simulink library "Yaw_System_Lib"  (Simulink 7.9)
settings: Solver=ode45  StartTime=0.0  StopTime=10.0  RelTol=1e-3
undefined symbols (not defined in the file): WT_Params
libraries: mblibv1 x45, Yaw_Actuation_Lib x3, Yaw_System_Lib x1
(part 1 of 2)
Description:
  | Copyright 2011 MathWorks, Inc.
settings Model: Creator=smiller  LastModifiedBy=smiller

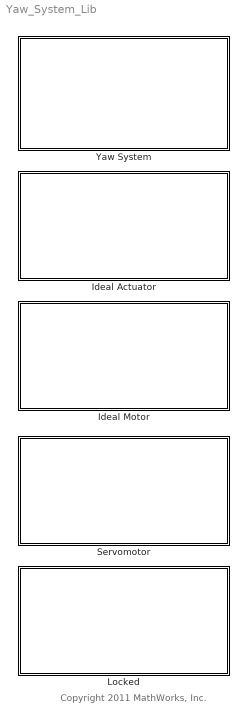
== system Yaw_System_Lib ==
  note: Copyright 2011 MathWorks, Inc.
  Ideal Actuator : Subsystem
      mask Display: image(imread('Yaw_Ideal_Actuator_System_IMAGE.jpg'));
  Ideal Motor : Subsystem
      mask Display: image(imread('Yaw_Ideal_Motor_System_IMAGE.jpg'));
  Locked : Subsystem
      mask Display: image(imread('Yaw_Locked_System_IMAGE.jpg'));
  Servomotor : Subsystem
      mask Display: image(imread('Yaw_Servomotor_System_IMAGE.jpg'));
  Yaw System : Subsystem  BlockChoice=Ideal Actuator
      settings: TemplateBlock=self  MemberBlocks=Ideal Actuator,Ideal Motor,Locked,Servomotor

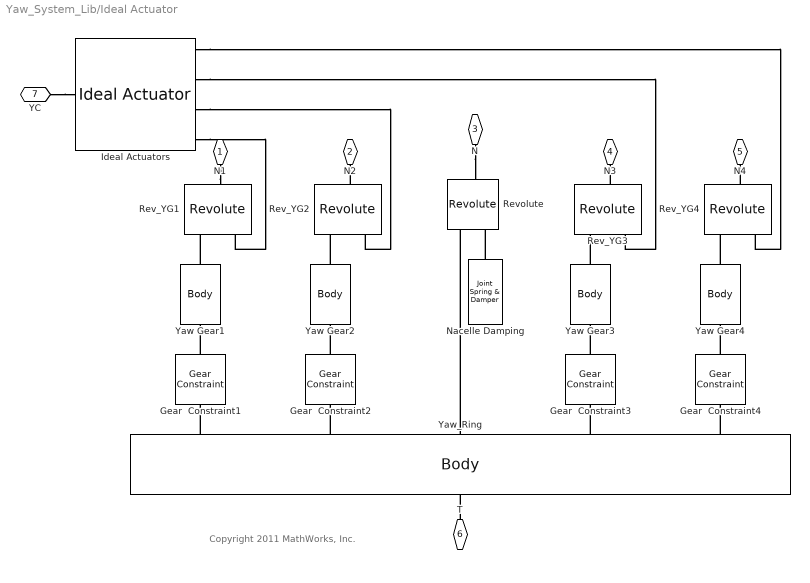
== system Yaw_System_Lib/Ideal Actuator ==
  note: Copyright 2011 MathWorks, Inc.
  Gear  Constraint{1..4} (4 alike) : mblibv1/Constraints &  Drivers/Gear Constraint  PhysicalDomain=mechanical  SubClassName=Unknown  LeftPortType=blob  RightPortType=blob  LConnTagsString=__newl0  RConnTagsString=__newr0  UpdateFromCAD=off  DialogClass=GearConstraint  NumSAPorts=0  BaseRadius=WT_Params.Yaw_Actuator.yaw_ring_diameter/2  BaseRadiusUnits=m  FollowerRadius=WT_Params.Yaw_Actuator.yaw_gear_diameter/2  FollowerRadiusUnits=m
  Ideal Actuators : Yaw_Actuation_Lib/Ideal Actuator  SystemSampleTime=-1
  Nacelle Damping : mblibv1/Force  Elements/Joint Spring & Damper  SystemSampleTime=-1  UpdateFromCAD=off  DialogClass=JointSpringDamper  JFEParameters=P1$false$0$0$0$m$m/s$N$deg$deg/s$N*m#P2$false$0$0$0$m$m/s$N$deg$deg/s$N*m#P3$false$0$0$0$m$m/s$N$deg$deg/s$N*m#R1$true$0$WT_Params.Nacelle.damping$0$m$m/s$N$deg$deg/s$N*m#R2$false$0$0$0$m$m/s$N$deg$deg/s$N*m#R3$false$0$0$0$m$m/s$N$deg$deg/s$N*m#S$false$0$0$0$m$m/s$N$deg$deg/s$N*m
  Rev_YG{1..4} (4 alike) : mblibv1/Joints/Revolute  LConnTagsString=__newl0|SA1  RConnTagsString=__newr0  UpdateFromCAD=off  NumSAPorts=1  CutJoint=off  MarkAsCut=off  Primitives=prismatic  PrimitiveProps=R1$Base$[0 1 0]$revolute  DialogClass=JointBlock  R1Axis=[0 1 0]
  Revolute : mblibv1/Joints/Revolute  LConnTagsString=__newl0|SA1  RConnTagsString=__newr0  UpdateFromCAD=off  NumSAPorts=1  CutJoint=off  MarkAsCut=off  Primitives=prismatic  PrimitiveProps=R1$Base$[0 1 0]$revolute  DialogClass=JointBlock  R1Axis=[0 1 0]
  Yaw Gear{1..4} (4 alike) : mblibv1/Bodies/Body  PhysicalDomain=mechanical  SubClassName=Unknown  LeftPortType=workingframe  RightPortType=workingframe  LConnTagsString=CG  RConnTagsString=CS1  UpdateFromCAD=off  DialogClass=MechanicalBodyBlock  Mass=1  MassUnits=kg  InertiaUnits=kg*m^2  Inertia=eye(3)  Shape=Cylinder  ShapeDims=[1 1]  ShapeUnits=m  ShapeUse=false  Density=1  DensityUnits=kg/m^3  DensityUse=false  GraphicsMode=MACHINE_DEFAULT  BodyColorSelMode=COLORPALETTE  BodyColor=[0 0 1]  AttachedToCS=CG  CG=Left$CG$[0 0 0]$ADJOINING$ADJOINING$m$[0 0 0]$Euler X-Y-Z$deg$ADJOINING$true$none  WorkingFrames=Right$CS1$[0 0 0]$CG$CG$m$[0 0 0]$Euler X-Y-Z$deg$CG$true$none#Right$CS5$[0 0 0]$CG$CG$m$[0 0 0]$Euler X-Y-Z$deg$CG$false$none#Right$CS7$[WT_Params.Yaw_Actuator.yaw_gear_diameter/2*cos(0) -0.5*WT_Params.Yaw_Actuator.yaw_gear_thickness WT_Params.Yaw_Actuator.yaw_gear_diameter/2*sin(0)]$CG$CG$m$[0 0 0]$Euler X-Y-Z$deg$CG$false$none#Right$CS17$[WT_Params.Yaw_Actuator.yaw_gear_diameter/2*cos(0) 0.5*WT_Params.Yaw_Actuator.yaw_gear_thickness WT_Params.Yaw_Actuator.yaw_gear_diameter/2*sin(0)]$CG$CG$m$[0 0 0]$Euler X-Y-Z$deg$CG$false$none#Right$CS8$[WT_Params.Yaw_Actuator.yaw_gear_diameter/2*cos(0.2*pi) -0.5*WT_Params.Yaw_Actuator.yaw_gear_thickness WT_Params.Yaw_Actuator.yaw_gear_diameter/2*sin(0.2*pi)]$CG$CG$m$[0 0 0]$Euler X-Y-Z$deg$CG$false$none#Right$CS18$[WT_Params.Yaw_Actuator.yaw_gear_diameter/2*cos(0.2*pi) 0.5*WT_Params.Yaw_Actuator.yaw_gear_thickness WT_Params.Yaw_Actuator.yaw_gear_diameter/2*sin(0.2*pi)]$CG$CG$m$[0 0 0]$Euler X-Y-Z$deg$CG$false$none#Right$CS9$[WT_Params.Yaw_Actuator.yaw_gear_diameter/2*cos(0.4*pi) -0.5*WT_Params.Yaw_Actuator.yaw_gear_thickness WT_Params.Yaw_Actuator.yaw_gear_diameter/2*sin(0.4*pi)]$CG$CG$m$[0 0 0]$Euler X-Y-Z$deg$CG$false$none#Right$CS19$[WT_Params.Yaw_Actuator.yaw_gear_diameter/2*cos(0.4*pi) 0.5*WT_Params.Yaw_Actuator.yaw_gear_thickness WT_Params.Yaw_Actuator.yaw_gear_diameter/2*sin(0.4*pi)]$CG$CG$m$[0 0 0]$Euler X-Y-Z$deg$CG$false$none#Right$CS10$[WT_Params.Yaw_Actuator.yaw_gear_diameter/2*cos(0.6*pi) -0.5*WT_Params.Yaw_Actuator.yaw_gear_thickness WT_Params.Yaw_Actuator.yaw_gear_diameter/2*sin(0.6*pi)]$CG$CG$m$[0 0 0]$Euler X-Y-Z$deg$CG$false$none#Right$CS20$[WT_Params.Yaw_Actuator.yaw_gear_diameter/2*cos(0.6*pi) 0.5*WT_Params.Yaw_Actuator.yaw_gear_thickness WT_Params.Yaw_Actuator.yaw_gear_diameter/2*sin(0.6*pi)]$CG$CG$m$[0 0 0]$Euler X-Y-Z$deg$CG$false$none#Right$CS11$[WT_Params.Yaw_Actuator.yaw_gear_diameter/2*cos(0.8*pi) -0.5*WT_Params.Yaw_Actuator.yaw_gear_thickness WT_Params.Yaw_Actuator.yaw_gear_diameter/2*sin(0.8*pi)]$CG$CG$m$[0 0 0]$Euler X-Y-Z$deg$CG$false$none#Right$CS21$[WT_Params.Yaw_Actuator.yaw_gear_diameter/2*cos(0.8*pi) 0.5*WT_Params.Yaw_Actuator.yaw_gear_thickness WT_Params.Yaw_Actuator.yaw_gear_diameter/2*sin(0.8*pi)]$CG$CG$m$[0 0 0]$Euler X-Y-Z$deg$CG$false$none#Right$CS12$[WT_Params.Yaw_Actuator.yaw_gear_diameter/2*cos(1.0*pi) -0.5*WT_Params.Yaw_Actuator.yaw_gear_thickness WT_Params.Yaw_Actuator.yaw_gear_diameter/2*sin(1.0*pi)]$CG$CG$m$[0 0 0]$Euler X-Y-Z$deg$CG$false$none#Right$CS22$[WT_Params.Yaw_Actuator.yaw_gear_diameter/2*cos(1.0*pi) 0.5*WT_Params.Yaw_Actuator.yaw_gear_thickness WT_Params.Yaw_Actuator.yaw_gear_diameter/2*sin(1.0*pi)]$CG$CG$m$[0 0 0]$Euler X-Y-Z$deg$CG$false$none#Right$CS13$[WT_Params.Yaw_Actuator.yaw_gear_diameter/2*cos(1.2*pi) -0.5*WT_Params.Yaw_Actuator.yaw_gear_thickness WT_Params.Yaw_Actuator.yaw_gear_diameter/2*sin(1.2*pi)]$CG$CG$m$[0 0 0]$Euler X-Y-Z$deg$CG$false$none#Right$CS23$[WT_Params.Yaw_Actuator.yaw_gear_diameter/2*cos(1.2*pi) 0.5*WT_Params.Yaw_Actuator.yaw_gear_thickness WT_Params.Yaw_Actuator.yaw_gear_diameter/2*sin(1.2*pi)]$CG$CG$m$[0 0 0]$Euler X-Y-Z$deg$CG$false$none#Right$CS14$[WT_Params.Yaw_Actuator.yaw_gear_diameter/2*cos(1.4*pi) -0.5*WT_Params.Yaw_Actuator.yaw_gear_thickness WT_Params.Yaw_Actuator.yaw_gear_diameter/2*sin(1.4*pi)]$CG$CG$m$[0 0 0]$Euler X-Y-Z$deg$CG$false$none#Right$CS24$[WT_Params.Yaw_Actuator.yaw_gear_diameter/2*cos(1.4*pi) 0.5*WT_Params.Yaw_Actuator.yaw_gear_thickness WT_Params.Yaw_Actuator.yaw_gear_diameter/2*sin(1.4*pi)]$CG$CG$m$[0 0 0]$Euler X-Y-Z$deg$CG$false$none#Right$CS15$[WT_Params.Yaw_Actuator.yaw_gear_diameter/2*cos(1.6*pi) -0.5*WT_Params.Yaw_Actuator.yaw_gear_thickness WT_Params.Yaw_Actuator.yaw_gear_diameter/2*sin(1.6*pi)]$CG$CG$m$[0 0 0]$Euler X-Y-Z$deg$CG$false$none#Right$CS25$[WT_Params.Yaw_Actuator.yaw_gear_diameter/2*cos(1.6*pi) 0.5*WT_Params.Yaw_Actuator.yaw_gear_thickness WT_Params.Yaw_Actuator.yaw_gear_diameter/2*sin(1.6*pi)]$CG$CG$m$[0 0 0]$Euler X-Y-Z$deg$CG$false$none#Right$CS16$[WT_Params.Yaw_Actuator.yaw_gear_diameter/2*cos(1.8*pi) -0.5*WT_Params.Yaw_Actuator.yaw_gear_thickness WT_Params.Yaw_Actuator.yaw_gear_diameter/2*sin(1.8*pi)]$CG$CG$m$[0 0 0]$Euler X-Y-Z$deg$CG$false$none#Right$CS26$[WT_Params.Yaw_Actuator.yaw_gear_diameter/2*cos(1.8*pi) 0.5*WT_Params.Yaw_Actuator.yaw_gear_thickness WT_Params.Yaw_Actuator.yaw_gear_diameter/2*sin(1.8*pi)]$CG$CG$m$[0 0 0]$Euler X-Y-Z$deg$CG$false$none  CGPos=[0 0 0]  CGRot=[0 0 0]  CS0Pos=[]  CS0Rot=[]  CS1Pos=[0 0 0]  CS1Rot=[0 0 0]  CS2Pos=[]  CS2Rot=[]  CS3Pos=[]  CS3Rot=[]  CS4Pos=[]  CS4Rot=[]  CS5Pos=[0 0 0]  CS5Rot=[0 0 0]  CS6Pos=[]  CS6Rot=[]  CS7Pos=[WT_Params.Yaw_Actuator.yaw_gear_diameter/2*cos(0) -0.5*WT_Params.Yaw_Actuator.yaw_gear_thickness WT_Params.Yaw_Actuator.yaw_gear_diameter/2*sin(0)]  CS7Rot=[0 0 0]  CS8Pos=[WT_Params.Yaw_Actuator.yaw_gear_diameter/2*cos(0.2*pi) -0.5*WT_Params.Yaw_Actuator.yaw_gear_thickness WT_Params.Yaw_Actuator.yaw_gear_diameter/2*sin(0.2*pi)]  CS8Rot=[0 0 0]  CS9Pos=[WT_Params.Yaw_Actuator.yaw_gear_diameter/2*cos(0.4*pi) -0.5*WT_Params.Yaw_Actuator.yaw_gear_thickness WT_Params.Yaw_Actuator.yaw_gear_diameter/2*sin(0.4*pi)]  CS9Rot=[0 0 0]  CS10Pos=[WT_Params.Yaw_Actuator.yaw_gear_diameter/2*cos(0.6*pi) -0.5*WT_Params.Yaw_Actuator.yaw_gear_thickness WT_Params.Yaw_Actuator.yaw_gear_diameter/2*sin(0.6*pi)]  CS10Rot=[0 0 0]  CS11Pos=[WT_Params.Yaw_Actuator.yaw_gear_diameter/2*cos(0.8*pi) -0.5*WT_Params.Yaw_Actuator.yaw_gear_thickness WT_Params.Yaw_Actuator.yaw_gear_diameter/2*sin(0.8*pi)]  CS11Rot=[0 0 0]  CS12Pos=[WT_Params.Yaw_Actuator.yaw_gear_diameter/2*cos(1.0*pi) -0.5*WT_Params.Yaw_Actuator.yaw_gear_thickness WT_Params.Yaw_Actuator.yaw_gear_diameter/2*sin(1.0*pi)]  CS12Rot=[0 0 0]  CS13Pos=[WT_Params.Yaw_Actuator.yaw_gear_diameter/2*cos(1.2*pi) -0.5*WT_Params.Yaw_Actuator.yaw_gear_thickness WT_Params.Yaw_Actuator.yaw_gear_diameter/2*sin(1.2*pi)]  CS13Rot=[0 0 0]  CS14Pos=[WT_Params.Yaw_Actuator.yaw_gear_diameter/2*cos(1.4*pi) -0.5*WT_Params.Yaw_Actuator.yaw_gear_thickness WT_Params.Yaw_Actuator.yaw_gear_diameter/2*sin(1.4*pi)]  CS14Rot=[0 0 0]  CS15Pos=[WT_Params.Yaw_Actuator.yaw_gear_diameter/2*cos(1.6*pi) -0.5*WT_Params.Yaw_Actuator.yaw_gear_thickness WT_Params.Yaw_Actuator.yaw_gear_diameter/2*sin(1.6*pi)]  CS15Rot=[0 0 0]  CS16Pos=[WT_Params.Yaw_Actuator.yaw_gear_diameter/2*cos(1.8*pi) -0.5*WT_Params.Yaw_Actuator.yaw_gear_thickness WT_Params.Yaw_Actuator.yaw_gear_diameter/2*sin(1.8*pi)]  CS16Rot=[0 0 0]  CS17Pos=[WT_Params.Yaw_Actuator.yaw_gear_diameter/2*cos(0) 0.5*WT_Params.Yaw_Actuator.yaw_gear_thickness WT_Params.Yaw_Actuator.yaw_gear_diameter/2*sin(0)]  CS17Rot=[0 0 0]  CS18Pos=[WT_Params.Yaw_Actuator.yaw_gear_diameter/2*cos(0.2*pi) 0.5*WT_Params.Yaw_Actuator.yaw_gear_thickness WT_Params.Yaw_Actuator.yaw_gear_diameter/2*sin(0.2*pi)]  CS18Rot=[0 0 0]  CS19Pos=[WT_Params.Yaw_Actuator.yaw_gear_diameter/2*cos(0.4*pi) 0.5*WT_Params.Yaw_Actuator.yaw_gear_thickness WT_Params.Yaw_Actuator.yaw_gear_diameter/2*sin(0.4*pi)]  CS19Rot=[0 0 0]  CS20Pos=[WT_Params.Yaw_Actuator.yaw_gear_diameter/2*cos(0.6*pi) 0.5*WT_Params.Yaw_Actuator.yaw_gear_thickness WT_Params.Yaw_Actuator.yaw_gear_diameter/2*sin(0.6*pi)]  CS20Rot=[0 0 0]
  Yaw_Ring : mblibv1/Bodies/Body  LConnTagsString=CS3|CS4|CS2|CS6|CS27  RConnTagsString=CS1  UpdateFromCAD=off  DialogClass=MechanicalBodyBlock  Mass=1  MassUnits=kg  InertiaUnits=kg*m^2  Inertia=eye(3)  Shape=Cylinder  ShapeDims=[1 1]  ShapeUnits=m  ShapeUse=false  Density=1  DensityUnits=kg/m^3  DensityUse=false  GraphicsMode=MACHINE_DEFAULT  BodyColorSelMode=COLORPALETTE  BodyColor=[0.74902 0.74902 0]  AttachedToCS=CG  CG=Left$CG$[0 0 0]$CS1$CS1$m$[0 0 0]$Euler X-Y-Z$deg$CS1$false$none  WorkingFrames=Left$CS3$[0 0 0]$CS1$CS1$m$[0 0 0]$Euler X-Y-Z$deg$CS1$true$none#Left$CS4$[0 0 0]$CS1$CS1$m$[0 0 0]$Euler X-Y-Z$deg$CS1$true$none#Left$CS2$[0 0 0]$CS1$CS1$m$[0 0 0]$Euler X-Y-Z$deg$CS1$true$none#Left$CS6$[0 0 0]$CS1$CS1$m$[0 0 0]$Euler X-Y-Z$deg$CS1$true$none#Left$CS27$[0 0 0]$CS1$CS1$m$[0 0 0]$Euler X-Y-Z$deg$CS1$true$none#Right$CS1$[0 0 0]$Adjoining$Adjoining$m$[0 0 0]$Euler X-Y-Z$deg$Adjoining$true$none#Right$CS5$[0 0 0]$CG$CG$m$[0 0 0]$Euler X-Y-Z$deg$CG$false$none#Right$CS7$[WT_Params.Yaw_Actuator.yaw_ring_diameter/2*cos(0) -0.5*WT_Params.Yaw_Actuator.yaw_ring_thickness WT_Params.Yaw_Actuator.yaw_ring_diameter/2*sin(0)]$CG$CG$m$[0 0 0]$Euler X-Y-Z$deg$CG$false$none#Right$CS17$[WT_Params.Yaw_Actuator.yaw_ring_diameter/2*cos(0) 0.5*WT_Params.Yaw_Actuator.yaw_gear_thickness WT_Params.Yaw_Actuator.yaw_ring_diameter/2*sin(0)]$CG$CG$m$[0 0 0]$Euler X-Y-Z$deg$CG$false$none#Right$CS8$[WT_Params.Yaw_Actuator.yaw_ring_diameter/2*cos(0.2*pi) -0.5*WT_Params.Yaw_Actuator.yaw_gear_thickness WT_Params.Yaw_Actuator.yaw_ring_diameter/2*sin(0.2*pi)]$CG$CG$m$[0 0 0]$Euler X-Y-Z$deg$CG$false$none#Right$CS18$[WT_Params.Yaw_Actuator.yaw_ring_diameter/2*cos(0.2*pi) 0.5*WT_Params.Yaw_Actuator.yaw_ring_thickness WT_Params.Yaw_Actuator.yaw_ring_diameter/2*sin(0.2*pi)]$CG$CG$m$[0 0 0]$Euler X-Y-Z$deg$CG$false$none#Right$CS9$[WT_Params.Yaw_Actuator.yaw_ring_diameter/2*cos(0.4*pi) -0.5*WT_Params.Yaw_Actuator.yaw_ring_thickness WT_Params.Yaw_Actuator.yaw_ring_diameter/2*sin(0.4*pi)]$CG$CG$m$[0 0 0]$Euler X-Y-Z$deg$CG$false$none#Right$CS19$[WT_Params.Yaw_Actuator.yaw_ring_diameter/2*cos(0.4*pi) 0.5*WT_Params.Yaw_Actuator.yaw_ring_thickness WT_Params.Yaw_Actuator.yaw_ring_diameter/2*sin(0.4*pi)]$CG$CG$m$[0 0 0]$Euler X-Y-Z$deg$CG$false$none#Right$CS10$[WT_Params.Yaw_Actuator.yaw_ring_diameter/2*cos(0.6*pi) -0.5*WT_Params.Yaw_Actuator.yaw_ring_thickness WT_Params.Yaw_Actuator.yaw_ring_diameter/2*sin(0.6*pi)]$CG$CG$m$[0 0 0]$Euler X-Y-Z$deg$CG$false$none#Right$CS20$[WT_Params.Yaw_Actuator.yaw_ring_diameter/2*cos(0.6*pi) 0.5*WT_Params.Yaw_Actuator.yaw_ring_thickness WT_Params.Yaw_Actuator.yaw_ring_diameter/2*sin(0.6*pi)]$CG$CG$m$[0 0 0]$Euler X-Y-Z$deg$CG$false$none#Right$CS11$[WT_Params.Yaw_Actuator.yaw_ring_diameter/2*cos(0.8*pi) -0.5*WT_Params.Yaw_Actuator.yaw_ring_thickness WT_Params.Yaw_Actuator.yaw_ring_diameter/2*sin(0.8*pi)]$CG$CG$m$[0 0 0]$Euler X-Y-Z$deg$CG$false$none#Right$CS21$[WT_Params.Yaw_Actuator.yaw_ring_diameter/2*cos(0.8*pi) 0.5*WT_Params.Yaw_Actuator.yaw_ring_thickness WT_Params.Yaw_Actuator.yaw_ring_diameter/2*sin(0.8*pi)]$CG$CG$m$[0 0 0]$Euler X-Y-Z$deg$CG$false$none#Right$CS12$[WT_Params.Yaw_Actuator.yaw_ring_diameter/2*cos(1.0*pi) -0.5*WT_Params.Yaw_Actuator.yaw_ring_thickness WT_Params.Yaw_Actuator.yaw_gear_diameter/2*sin(1.0*pi)]$CG$CG$m$[0 0 0]$Euler X-Y-Z$deg$CG$false$none#Right$CS22$[WT_Params.Yaw_Actuator.yaw_gear_diameter/2*cos(1.0*pi) 0.5*WT_Params.Yaw_Actuator.yaw_ring_thickness WT_Params.Yaw_Actuator.yaw_ring_diameter/2*sin(1.0*pi)]$CG$CG$m$[0 0 0]$Euler X-Y-Z$deg$CG$false$none#Right$CS13$[WT_Params.Yaw_Actuator.yaw_ring_diameter/2*cos(1.2*pi) -0.5*WT_Params.Yaw_Actuator.yaw_ring_thickness WT_Params.Yaw_Actuator.yaw_ring_diameter/2*sin(1.2*pi)]$CG$CG$m$[0 0 0]$Euler X-Y-Z$deg$CG$false$none#Right$CS23$[WT_Params.Yaw_Actuator.yaw_ring_diameter/2*cos(1.2*pi) 0.5*WT_Params.Yaw_Actuator.yaw_ring_thickness WT_Params.Yaw_Actuator.yaw_ring_diameter/2*sin(1.2*pi)]$CG$CG$m$[0 0 0]$Euler X-Y-Z$deg$CG$false$none#Right$CS14$[WT_Params.Yaw_Actuator.yaw_ring_diameter/2*cos(1.4*pi) -0.5*WT_Params.Yaw_Actuator.yaw_gear_thickness WT_Params.Yaw_Actuator.yaw_ring_diameter/2*sin(1.4*pi)]$CG$CG$m$[0 0 0]$Euler X-Y-Z$deg$CG$false$none#Right$CS24$[WT_Params.Yaw_Actuator.yaw_ring_diameter/2*cos(1.4*pi) 0.5*WT_Params.Yaw_Actuator.yaw_ring_thickness WT_Params.Yaw_Actuator.yaw_ring_diameter/2*sin(1.4*pi)]$CG$CG$m$[0 0 0]$Euler X-Y-Z$deg$CG$false$none#Right$CS15$[WT_Params.Yaw_Actuator.yaw_ring_diameter/2*cos(1.6*pi) -0.5*WT_Params.Yaw_Actuator.yaw_ring_thickness WT_Params.Yaw_Actuator.yaw_ring_diameter/2*sin(1.6*pi)]$CG$CG$m$[0 0 0]$Euler X-Y-Z$deg$CG$false$none#Right$CS25$[WT_Params.Yaw_Actuator.yaw_ring_diameter/2*cos(1.6*pi) 0.5*WT_Params.Yaw_Actuator.yaw_ring_thickness WT_Params.Yaw_Actuator.yaw_ring_diameter/2*sin(1.6*pi)]$CG$CG$m$[0 0 0]$Euler X-Y-Z$deg$CG$false$none#Right$CS16$[WT_Params.Yaw_Actuator.yaw_ring_diameter/2*cos(1.8*pi) -0.5*WT_Params.Yaw_Actuator.yaw_ring_thickness WT_Params.Yaw_Actuator.yaw_ring_diameter/2*sin(1.8*pi)]$CG$CG$m$[0 0 0]$Euler X-Y-Z$deg$CG$false$none#Right$CS26$[WT_Params.Yaw_Actuator.yaw_ring_diameter/2*cos(1.8*pi) 0.5*WT_Params.Yaw_Actuator.yaw_ring_thickness WT_Params.Yaw_Actuator.yaw_ring_diameter/2*sin(1.8*pi)]$CG$CG$m$[0 0 0]$Euler X-Y-Z$deg$CG$false$none  CGPos=[0 0 0]  CGRot=[0 0 0]  CS0Pos=[]  CS0Rot=[]  CS1Pos=[0 0 0]  CS1Rot=[0 0 0]  CS2Pos=[0 0 0]  CS2Rot=[0 0 0]  CS3Pos=[0 0 0]  CS3Rot=[0 0 0]  CS4Pos=[0 0 0]  CS4Rot=[0 0 0]  CS5Pos=[0 0 0]  CS5Rot=[0 0 0]  CS6Pos=[0 0 0]  CS6Rot=[0 0 0]  CS7Pos=[WT_Params.Yaw_Actuator.yaw_ring_diameter/2*cos(0) -0.5*WT_Params.Yaw_Actuator.yaw_ring_thickness WT_Params.Yaw_Actuator.yaw_ring_diameter/2*sin(0)]  CS7Rot=[0 0 0]  CS8Pos=[WT_Params.Yaw_Actuator.yaw_ring_diameter/2*cos(0.2*pi) -0.5*WT_Params.Yaw_Actuator.yaw_gear_thickness WT_Params.Yaw_Actuator.yaw_ring_diameter/2*sin(0.2*pi)]  CS8Rot=[0 0 0]  CS9Pos=[WT_Params.Yaw_Actuator.yaw_ring_diameter/2*cos(0.4*pi) -0.5*WT_Params.Yaw_Actuator.yaw_ring_thickness WT_Params.Yaw_Actuator.yaw_ring_diameter/2*sin(0.4*pi)]  CS9Rot=[0 0 0]  CS10Pos=[WT_Params.Yaw_Actuator.yaw_ring_diameter/2*cos(0.6*pi) -0.5*WT_Params.Yaw_Actuator.yaw_ring_thickness WT_Params.Yaw_Actuator.yaw_ring_diameter/2*sin(0.6*pi)]  CS10Rot=[0 0 0]  CS11Pos=[WT_Params.Yaw_Actuator.yaw_ring_diameter/2*cos(0.8*pi) -0.5*WT_Params.Yaw_Actuator.yaw_ring_thickness WT_Params.Yaw_Actuator.yaw_ring_diameter/2*sin(0.8*pi)]  CS11Rot=[0 0 0]  CS12Pos=[WT_Params.Yaw_Actuator.yaw_ring_diameter/2*cos(1.0*pi) -0.5*WT_Params.Yaw_Actuator.yaw_ring_thickness WT_Params.Yaw_Actuator.yaw_gear_diameter/2*sin(1.0*pi)]  CS12Rot=[0 0 0]  CS13Pos=[WT_Params.Yaw_Actuator.yaw_ring_diameter/2*cos(1.2*pi) -0.5*WT_Params.Yaw_Actuator.yaw_ring_thickness WT_Params.Yaw_Actuator.yaw_ring_diameter/2*sin(1.2*pi)]  CS13Rot=[0 0 0]  CS14Pos=[WT_Params.Yaw_Actuator.yaw_ring_diameter/2*cos(1.4*pi) -0.5*WT_Params.Yaw_Actuator.yaw_gear_thickness WT_Params.Yaw_Actuator.yaw_ring_diameter/2*sin(1.4*pi)]  CS14Rot=[0 0 0]  CS15Pos=[WT_Params.Yaw_Actuator.yaw_ring_diameter/2*cos(1.6*pi) -0.5*WT_Params.Yaw_Actuator.yaw_ring_thickness WT_Params.Yaw_Actuator.yaw_ring_diameter/2*sin(1.6*pi)]  CS15Rot=[0 0 0]  CS16Pos=[WT_Params.Yaw_Actuator.yaw_ring_diameter/2*cos(1.8*pi) -0.5*WT_Params.Yaw_Actuator.yaw_ring_thickness WT_Params.Yaw_Actuator.yaw_ring_diameter/2*sin(1.8*pi)]  CS16Rot=[0 0 0]  CS17Pos=[WT_Params.Yaw_Actuator.yaw_ring_diameter/2*cos(0) 0.5*WT_Params.Yaw_Actuator.yaw_gear_thickness WT_Params.Yaw_Actuator.yaw_ring_diameter/2*sin(0)]  CS17Rot=[0 0 0]  CS18Pos=[WT_Params.Yaw_Actuator.yaw_ring_diameter/2*cos(0.2*pi) 0.5*WT_Params.Yaw_Actuator.yaw_ring_thickness WT_Params.Yaw_Actuator.yaw_ring_diameter/2*sin(0.2*pi)]  CS18Rot=[0 0 0]  CS19Pos=[WT_Params.Yaw_Actuator.yaw_ring_diameter/2*cos(0.4*pi) 0.5*WT_Params.Yaw_Actuator.yaw_ring_thickness WT_Params.Yaw_Actuator.yaw_ring_diameter/2*sin(0.4*pi)]  CS19Rot=[0 0 0]  CS20Pos=[WT_Params.Yaw_Actuator.yaw_ring_diameter/2*cos(0.6*pi) 0.5*WT_Params.Yaw_Actuator.yaw_ring_thickness WT_Params.Yaw_Actuator.yaw_ring_diameter/2*sin(0.6*pi)]  CS20Rot=[0 0 0]
  N1 : PMIOPort  Port=1  Side=Right
  N2 : PMIOPort  Port=2  Side=Right
  N : PMIOPort  Port=3  Side=Right
  N3 : PMIOPort  Port=4  Side=Right
  N4 : PMIOPort  Port=5  Side=Right
  T : PMIOPort  Port=6  Side=Left
  YC : PMIOPort  Port=7  Side=Right
  connections:
  Gear  Constraint1/RConn1 -- Yaw Gear1/RConn1
  Yaw Gear1/LConn1 -- Rev_YG1/LConn1
  N1/RConn1 -- Rev_YG1/RConn1
  Gear  Constraint2/RConn1 -- Yaw Gear2/RConn1
  Yaw Gear2/LConn1 -- Rev_YG2/LConn1
  Rev_YG2/RConn1 -- N2/RConn1
  Gear  Constraint3/RConn1 -- Yaw Gear3/RConn1
  Yaw Gear3/LConn1 -- Rev_YG3/LConn1
  Rev_YG3/RConn1 -- N3/RConn1
  Gear  Constraint4/RConn1 -- Yaw Gear4/RConn1
  Yaw_Ring/LConn5 -- Gear  Constraint4/LConn1
  Rev_YG4/RConn1 -- N4/RConn1
  Yaw Gear4/LConn1 -- Rev_YG4/LConn1
  YC/RConn1 -- Ideal Actuators/LConn1
  Ideal Actuators/RConn4 -- Rev_YG1/LConn2
  Ideal Actuators/RConn3 -- Rev_YG2/LConn2
  Ideal Actuators/RConn2 -- Rev_YG3/LConn2
  Ideal Actuators/RConn1 -- Rev_YG4/LConn2
  Nacelle Damping/LConn1 -- Revolute/LConn2
  N/RConn1 -- Revolute/RConn1
  Yaw_Ring/LConn3 -- Revolute/LConn1
  Yaw_Ring/LConn1 -- Gear  Constraint1/LConn1
  Yaw_Ring/LConn2 -- Gear  Constraint2/LConn1
  Yaw_Ring/LConn4 -- Gear  Constraint3/LConn1
  T/RConn1 -- Yaw_Ring/RConn1

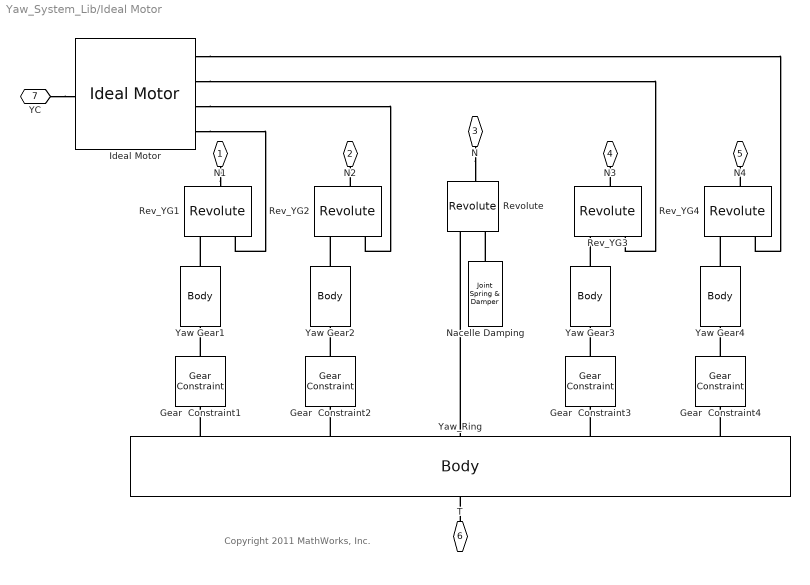
== system Yaw_System_Lib/Ideal Motor ==
  note: Copyright 2011 MathWorks, Inc.
  Gear  Constraint{1..4} (4 alike) : mblibv1/Constraints &  Drivers/Gear Constraint  PhysicalDomain=mechanical  SubClassName=Unknown  LeftPortType=blob  RightPortType=blob  LConnTagsString=__newl0  RConnTagsString=__newr0  UpdateFromCAD=off  DialogClass=GearConstraint  NumSAPorts=0  BaseRadius=WT_Params.Yaw_Actuator.yaw_ring_diameter/2  BaseRadiusUnits=m  FollowerRadius=WT_Params.Yaw_Actuator.yaw_gear_diameter/2  FollowerRadiusUnits=m
  Ideal Motor : Yaw_Actuation_Lib/Ideal Motor  SystemSampleTime=-1
  Nacelle Damping : mblibv1/Force  Elements/Joint Spring & Damper  SystemSampleTime=-1  UpdateFromCAD=off  DialogClass=JointSpringDamper  JFEParameters=P1$false$0$0$0$m$m/s$N$deg$deg/s$N*m#P2$false$0$0$0$m$m/s$N$deg$deg/s$N*m#P3$false$0$0$0$m$m/s$N$deg$deg/s$N*m#R1$true$0$WT_Params.Nacelle.damping$0$m$m/s$N$deg$deg/s$N*m#R2$false$0$0$0$m$m/s$N$deg$deg/s$N*m#R3$false$0$0$0$m$m/s$N$deg$deg/s$N*m#S$false$0$0$0$m$m/s$N$deg$deg/s$N*m
  Rev_YG{1..4} (4 alike) : mblibv1/Joints/Revolute  LConnTagsString=__newl0|SA1  RConnTagsString=__newr0  UpdateFromCAD=off  NumSAPorts=1  CutJoint=off  MarkAsCut=off  Primitives=prismatic  PrimitiveProps=R1$Base$[0 1 0]$revolute  DialogClass=JointBlock  R1Axis=[0 1 0]
  Revolute : mblibv1/Joints/Revolute  LConnTagsString=__newl0|SA1  RConnTagsString=__newr0  UpdateFromCAD=off  NumSAPorts=1  CutJoint=off  MarkAsCut=off  Primitives=prismatic  PrimitiveProps=R1$Base$[0 1 0]$revolute  DialogClass=JointBlock  R1Axis=[0 1 0]
  Yaw Gear{1..4} (4 alike) : mblibv1/Bodies/Body  PhysicalDomain=mechanical  SubClassName=Unknown  LeftPortType=workingframe  RightPortType=workingframe  LConnTagsString=CG  RConnTagsString=CS1  UpdateFromCAD=off  DialogClass=MechanicalBodyBlock  Mass=1  MassUnits=kg  InertiaUnits=kg*m^2  Inertia=eye(3)  Shape=Cylinder  ShapeDims=[1 1]  ShapeUnits=m  ShapeUse=false  Density=1  DensityUnits=kg/m^3  DensityUse=false  GraphicsMode=MACHINE_DEFAULT  BodyColorSelMode=COLORPALETTE  BodyColor=[0 0 1]  AttachedToCS=CG  CG=Left$CG$[0 0 0]$ADJOINING$ADJOINING$m$[0 0 0]$Euler X-Y-Z$deg$ADJOINING$true$none  WorkingFrames=Right$CS1$[0 0 0]$CG$CG$m$[0 0 0]$Euler X-Y-Z$deg$CG$true$none#Right$CS5$[0 0 0]$CG$CG$m$[0 0 0]$Euler X-Y-Z$deg$CG$false$none#Right$CS7$[WT_Params.Yaw_Actuator.yaw_gear_diameter/2*cos(0) -0.5*WT_Params.Yaw_Actuator.yaw_gear_thickness WT_Params.Yaw_Actuator.yaw_gear_diameter/2*sin(0)]$CG$CG$m$[0 0 0]$Euler X-Y-Z$deg$CG$false$none#Right$CS17$[WT_Params.Yaw_Actuator.yaw_gear_diameter/2*cos(0) 0.5*WT_Params.Yaw_Actuator.yaw_gear_thickness WT_Params.Yaw_Actuator.yaw_gear_diameter/2*sin(0)]$CG$CG$m$[0 0 0]$Euler X-Y-Z$deg$CG$false$none#Right$CS8$[WT_Params.Yaw_Actuator.yaw_gear_diameter/2*cos(0.2*pi) -0.5*WT_Params.Yaw_Actuator.yaw_gear_thickness WT_Params.Yaw_Actuator.yaw_gear_diameter/2*sin(0.2*pi)]$CG$CG$m$[0 0 0]$Euler X-Y-Z$deg$CG$false$none#Right$CS18$[WT_Params.Yaw_Actuator.yaw_gear_diameter/2*cos(0.2*pi) 0.5*WT_Params.Yaw_Actuator.yaw_gear_thickness WT_Params.Yaw_Actuator.yaw_gear_diameter/2*sin(0.2*pi)]$CG$CG$m$[0 0 0]$Euler X-Y-Z$deg$CG$false$none#Right$CS9$[WT_Params.Yaw_Actuator.yaw_gear_diameter/2*cos(0.4*pi) -0.5*WT_Params.Yaw_Actuator.yaw_gear_thickness WT_Params.Yaw_Actuator.yaw_gear_diameter/2*sin(0.4*pi)]$CG$CG$m$[0 0 0]$Euler X-Y-Z$deg$CG$false$none#Right$CS19$[WT_Params.Yaw_Actuator.yaw_gear_diameter/2*cos(0.4*pi) 0.5*WT_Params.Yaw_Actuator.yaw_gear_thickness WT_Params.Yaw_Actuator.yaw_gear_diameter/2*sin(0.4*pi)]$CG$CG$m$[0 0 0]$Euler X-Y-Z$deg$CG$false$none#Right$CS10$[WT_Params.Yaw_Actuator.yaw_gear_diameter/2*cos(0.6*pi) -0.5*WT_Params.Yaw_Actuator.yaw_gear_thickness WT_Params.Yaw_Actuator.yaw_gear_diameter/2*sin(0.6*pi)]$CG$CG$m$[0 0 0]$Euler X-Y-Z$deg$CG$false$none#Right$CS20$[WT_Params.Yaw_Actuator.yaw_gear_diameter/2*cos(0.6*pi) 0.5*WT_Params.Yaw_Actuator.yaw_gear_thickness WT_Params.Yaw_Actuator.yaw_gear_diameter/2*sin(0.6*pi)]$CG$CG$m$[0 0 0]$Euler X-Y-Z$deg$CG$false$none#Right$CS11$[WT_Params.Yaw_Actuator.yaw_gear_diameter/2*cos(0.8*pi) -0.5*WT_Params.Yaw_Actuator.yaw_gear_thickness WT_Params.Yaw_Actuator.yaw_gear_diameter/2*sin(0.8*pi)]$CG$CG$m$[0 0 0]$Euler X-Y-Z$deg$CG$false$none#Right$CS21$[WT_Params.Yaw_Actuator.yaw_gear_diameter/2*cos(0.8*pi) 0.5*WT_Params.Yaw_Actuator.yaw_gear_thickness WT_Params.Yaw_Actuator.yaw_gear_diameter/2*sin(0.8*pi)]$CG$CG$m$[0 0 0]$Euler X-Y-Z$deg$CG$false$none#Right$CS12$[WT_Params.Yaw_Actuator.yaw_gear_diameter/2*cos(1.0*pi) -0.5*WT_Params.Yaw_Actuator.yaw_gear_thickness WT_Params.Yaw_Actuator.yaw_gear_diameter/2*sin(1.0*pi)]$CG$CG$m$[0 0 0]$Euler X-Y-Z$deg$CG$false$none#Right$CS22$[WT_Params.Yaw_Actuator.yaw_gear_diameter/2*cos(1.0*pi) 0.5*WT_Params.Yaw_Actuator.yaw_gear_thickness WT_Params.Yaw_Actuator.yaw_gear_diameter/2*sin(1.0*pi)]$CG$CG$m$[0 0 0]$Euler X-Y-Z$deg$CG$false$none#Right$CS13$[WT_Params.Yaw_Actuator.yaw_gear_diameter/2*cos(1.2*pi) -0.5*WT_Params.Yaw_Actuator.yaw_gear_thickness WT_Params.Yaw_Actuator.yaw_gear_diameter/2*sin(1.2*pi)]$CG$CG$m$[0 0 0]$Euler X-Y-Z$deg$CG$false$none#Right$CS23$[WT_Params.Yaw_Actuator.yaw_gear_diameter/2*cos(1.2*pi) 0.5*WT_Params.Yaw_Actuator.yaw_gear_thickness WT_Params.Yaw_Actuator.yaw_gear_diameter/2*sin(1.2*pi)]$CG$CG$m$[0 0 0]$Euler X-Y-Z$deg$CG$false$none#Right$CS14$[WT_Params.Yaw_Actuator.yaw_gear_diameter/2*cos(1.4*pi) -0.5*WT_Params.Yaw_Actuator.yaw_gear_thickness WT_Params.Yaw_Actuator.yaw_gear_diameter/2*sin(1.4*pi)]$CG$CG$m$[0 0 0]$Euler X-Y-Z$deg$CG$false$none#Right$CS24$[WT_Params.Yaw_Actuator.yaw_gear_diameter/2*cos(1.4*pi) 0.5*WT_Params.Yaw_Actuator.yaw_gear_thickness WT_Params.Yaw_Actuator.yaw_gear_diameter/2*sin(1.4*pi)]$CG$CG$m$[0 0 0]$Euler X-Y-Z$deg$CG$false$none#Right$CS15$[WT_Params.Yaw_Actuator.yaw_gear_diameter/2*cos(1.6*pi) -0.5*WT_Params.Yaw_Actuator.yaw_gear_thickness WT_Params.Yaw_Actuator.yaw_gear_diameter/2*sin(1.6*pi)]$CG$CG$m$[0 0 0]$Euler X-Y-Z$deg$CG$false$none#Right$CS25$[WT_Params.Yaw_Actuator.yaw_gear_diameter/2*cos(1.6*pi) 0.5*WT_Params.Yaw_Actuator.yaw_gear_thickness WT_Params.Yaw_Actuator.yaw_gear_diameter/2*sin(1.6*pi)]$CG$CG$m$[0 0 0]$Euler X-Y-Z$deg$CG$false$none#Right$CS16$[WT_Params.Yaw_Actuator.yaw_gear_diameter/2*cos(1.8*pi) -0.5*WT_Params.Yaw_Actuator.yaw_gear_thickness WT_Params.Yaw_Actuator.yaw_gear_diameter/2*sin(1.8*pi)]$CG$CG$m$[0 0 0]$Euler X-Y-Z$deg$CG$false$none#Right$CS26$[WT_Params.Yaw_Actuator.yaw_gear_diameter/2*cos(1.8*pi) 0.5*WT_Params.Yaw_Actuator.yaw_gear_thickness WT_Params.Yaw_Actuator.yaw_gear_diameter/2*sin(1.8*pi)]$CG$CG$m$[0 0 0]$Euler X-Y-Z$deg$CG$false$none  CGPos=[0 0 0]  CGRot=[0 0 0]  CS0Pos=[]  CS0Rot=[]  CS1Pos=[0 0 0]  CS1Rot=[0 0 0]  CS2Pos=[]  CS2Rot=[]  CS3Pos=[]  CS3Rot=[]  CS4Pos=[]  CS4Rot=[]  CS5Pos=[0 0 0]  CS5Rot=[0 0 0]  CS6Pos=[]  CS6Rot=[]  CS7Pos=[WT_Params.Yaw_Actuator.yaw_gear_diameter/2*cos(0) -0.5*WT_Params.Yaw_Actuator.yaw_gear_thickness WT_Params.Yaw_Actuator.yaw_gear_diameter/2*sin(0)]  CS7Rot=[0 0 0]  CS8Pos=[WT_Params.Yaw_Actuator.yaw_gear_diameter/2*cos(0.2*pi) -0.5*WT_Params.Yaw_Actuator.yaw_gear_thickness WT_Params.Yaw_Actuator.yaw_gear_diameter/2*sin(0.2*pi)]  CS8Rot=[0 0 0]  CS9Pos=[WT_Params.Yaw_Actuator.yaw_gear_diameter/2*cos(0.4*pi) -0.5*WT_Params.Yaw_Actuator.yaw_gear_thickness WT_Params.Yaw_Actuator.yaw_gear_diameter/2*sin(0.4*pi)]  CS9Rot=[0 0 0]  CS10Pos=[WT_Params.Yaw_Actuator.yaw_gear_diameter/2*cos(0.6*pi) -0.5*WT_Params.Yaw_Actuator.yaw_gear_thickness WT_Params.Yaw_Actuator.yaw_gear_diameter/2*sin(0.6*pi)]  CS10Rot=[0 0 0]  CS11Pos=[WT_Params.Yaw_Actuator.yaw_gear_diameter/2*cos(0.8*pi) -0.5*WT_Params.Yaw_Actuator.yaw_gear_thickness WT_Params.Yaw_Actuator.yaw_gear_diameter/2*sin(0.8*pi)]  CS11Rot=[0 0 0]  CS12Pos=[WT_Params.Yaw_Actuator.yaw_gear_diameter/2*cos(1.0*pi) -0.5*WT_Params.Yaw_Actuator.yaw_gear_thickness WT_Params.Yaw_Actuator.yaw_gear_diameter/2*sin(1.0*pi)]  CS12Rot=[0 0 0]  CS13Pos=[WT_Params.Yaw_Actuator.yaw_gear_diameter/2*cos(1.2*pi) -0.5*WT_Params.Yaw_Actuator.yaw_gear_thickness WT_Params.Yaw_Actuator.yaw_gear_diameter/2*sin(1.2*pi)]  CS13Rot=[0 0 0]  CS14Pos=[WT_Params.Yaw_Actuator.yaw_gear_diameter/2*cos(1.4*pi) -0.5*WT_Params.Yaw_Actuator.yaw_gear_thickness WT_Params.Yaw_Actuator.yaw_gear_diameter/2*sin(1.4*pi)]  CS14Rot=[0 0 0]  CS15Pos=[WT_Params.Yaw_Actuator.yaw_gear_diameter/2*cos(1.6*pi) -0.5*WT_Params.Yaw_Actuator.yaw_gear_thickness WT_Params.Yaw_Actuator.yaw_gear_diameter/2*sin(1.6*pi)]  CS15Rot=[0 0 0]  CS16Pos=[WT_Params.Yaw_Actuator.yaw_gear_diameter/2*cos(1.8*pi) -0.5*WT_Params.Yaw_Actuator.yaw_gear_thickness WT_Params.Yaw_Actuator.yaw_gear_diameter/2*sin(1.8*pi)]  CS16Rot=[0 0 0]  CS17Pos=[WT_Params.Yaw_Actuator.yaw_gear_diameter/2*cos(0) 0.5*WT_Params.Yaw_Actuator.yaw_gear_thickness WT_Params.Yaw_Actuator.yaw_gear_diameter/2*sin(0)]  CS17Rot=[0 0 0]  CS18Pos=[WT_Params.Yaw_Actuator.yaw_gear_diameter/2*cos(0.2*pi) 0.5*WT_Params.Yaw_Actuator.yaw_gear_thickness WT_Params.Yaw_Actuator.yaw_gear_diameter/2*sin(0.2*pi)]  CS18Rot=[0 0 0]  CS19Pos=[WT_Params.Yaw_Actuator.yaw_gear_diameter/2*cos(0.4*pi) 0.5*WT_Params.Yaw_Actuator.yaw_gear_thickness WT_Params.Yaw_Actuator.yaw_gear_diameter/2*sin(0.4*pi)]  CS19Rot=[0 0 0]  CS20Pos=[WT_Params.Yaw_Actuator.yaw_gear_diameter/2*cos(0.6*pi) 0.5*WT_Params.Yaw_Actuator.yaw_gear_thickness WT_Params.Yaw_Actuator.yaw_gear_diameter/2*sin(0.6*pi)]  CS20Rot=[0 0 0]
  Yaw_Ring : mblibv1/Bodies/Body  LConnTagsString=CS3|CS4|CS2|CS6|CS27  RConnTagsString=CS1  UpdateFromCAD=off  DialogClass=MechanicalBodyBlock  Mass=1  MassUnits=kg  InertiaUnits=kg*m^2  Inertia=eye(3)  Shape=Cylinder  ShapeDims=[1 1]  ShapeUnits=m  ShapeUse=false  Density=1  DensityUnits=kg/m^3  DensityUse=false  GraphicsMode=MACHINE_DEFAULT  BodyColorSelMode=COLORPALETTE  BodyColor=[0.74902 0.74902 0]  AttachedToCS=CG  CG=Left$CG$[0 0 0]$CS1$CS1$m$[0 0 0]$Euler X-Y-Z$deg$CS1$false$none  WorkingFrames=Left$CS3$[0 0 0]$CS1$CS1$m$[0 0 0]$Euler X-Y-Z$deg$CS1$true$none#Left$CS4$[0 0 0]$CS1$CS1$m$[0 0 0]$Euler X-Y-Z$deg$CS1$true$none#Left$CS2$[0 0 0]$CS1$CS1$m$[0 0 0]$Euler X-Y-Z$deg$CS1$true$none#Left$CS6$[0 0 0]$CS1$CS1$m$[0 0 0]$Euler X-Y-Z$deg$CS1$true$none#Left$CS27$[0 0 0]$CS1$CS1$m$[0 0 0]$Euler X-Y-Z$deg$CS1$true$none#Right$CS1$[0 0 0]$Adjoining$Adjoining$m$[0 0 0]$Euler X-Y-Z$deg$Adjoining$true$none#Right$CS5$[0 0 0]$CG$CG$m$[0 0 0]$Euler X-Y-Z$deg$CG$false$none#Right$CS7$[WT_Params.Yaw_Actuator.yaw_ring_diameter/2*cos(0) -0.5*WT_Params.Yaw_Actuator.yaw_ring_thickness WT_Params.Yaw_Actuator.yaw_ring_diameter/2*sin(0)]$CG$CG$m$[0 0 0]$Euler X-Y-Z$deg$CG$false$none#Right$CS17$[WT_Params.Yaw_Actuator.yaw_ring_diameter/2*cos(0) 0.5*WT_Params.Yaw_Actuator.yaw_gear_thickness WT_Params.Yaw_Actuator.yaw_ring_diameter/2*sin(0)]$CG$CG$m$[0 0 0]$Euler X-Y-Z$deg$CG$false$none#Right$CS8$[WT_Params.Yaw_Actuator.yaw_ring_diameter/2*cos(0.2*pi) -0.5*WT_Params.Yaw_Actuator.yaw_gear_thickness WT_Params.Yaw_Actuator.yaw_ring_diameter/2*sin(0.2*pi)]$CG$CG$m$[0 0 0]$Euler X-Y-Z$deg$CG$false$none#Right$CS18$[WT_Params.Yaw_Actuator.yaw_ring_diameter/2*cos(0.2*pi) 0.5*WT_Params.Yaw_Actuator.yaw_ring_thickness WT_Params.Yaw_Actuator.yaw_ring_diameter/2*sin(0.2*pi)]$CG$CG$m$[0 0 0]$Euler X-Y-Z$deg$CG$false$none#Right$CS9$[WT_Params.Yaw_Actuator.yaw_ring_diameter/2*cos(0.4*pi) -0.5*WT_Params.Yaw_Actuator.yaw_ring_thickness WT_Params.Yaw_Actuator.yaw_ring_diameter/2*sin(0.4*pi)]$CG$CG$m$[0 0 0]$Euler X-Y-Z$deg$CG$false$none#Right$CS19$[WT_Params.Yaw_Actuator.yaw_ring_diameter/2*cos(0.4*pi) 0.5*WT_Params.Yaw_Actuator.yaw_ring_thickness WT_Params.Yaw_Actuator.yaw_ring_diameter/2*sin(0.4*pi)]$CG$CG$m$[0 0 0]$Euler X-Y-Z$deg$CG$false$none#Right$CS10$[WT_Params.Yaw_Actuator.yaw_ring_diameter/2*cos(0.6*pi) -0.5*WT_Params.Yaw_Actuator.yaw_ring_thickness WT_Params.Yaw_Actuator.yaw_ring_diameter/2*sin(0.6*pi)]$CG$CG$m$[0 0 0]$Euler X-Y-Z$deg$CG$false$none#Right$CS20$[WT_Params.Yaw_Actuator.yaw_ring_diameter/2*cos(0.6*pi) 0.5*WT_Params.Yaw_Actuator.yaw_ring_thickness WT_Params.Yaw_Actuator.yaw_ring_diameter/2*sin(0.6*pi)]$CG$CG$m$[0 0 0]$Euler X-Y-Z$deg$CG$false$none#Right$CS11$[WT_Params.Yaw_Actuator.yaw_ring_diameter/2*cos(0.8*pi) -0.5*WT_Params.Yaw_Actuator.yaw_ring_thickness WT_Params.Yaw_Actuator.yaw_ring_diameter/2*sin(0.8*pi)]$CG$CG$m$[0 0 0]$Euler X-Y-Z$deg$CG$false$none#Right$CS21$[WT_Params.Yaw_Actuator.yaw_ring_diameter/2*cos(0.8*pi) 0.5*WT_Params.Yaw_Actuator.yaw_ring_thickness WT_Params.Yaw_Actuator.yaw_ring_diameter/2*sin(0.8*pi)]$CG$CG$m$[0 0 0]$Euler X-Y-Z$deg$CG$false$none#Right$CS12$[WT_Params.Yaw_Actuator.yaw_ring_diameter/2*cos(1.0*pi) -0.5*WT_Params.Yaw_Actuator.yaw_ring_thickness WT_Params.Yaw_Actuator.yaw_gear_diameter/2*sin(1.0*pi)]$CG$CG$m$[0 0 0]$Euler X-Y-Z$deg$CG$false$none#Right$CS22$[WT_Params.Yaw_Actuator.yaw_gear_diameter/2*cos(1.0*pi) 0.5*WT_Params.Yaw_Actuator.yaw_ring_thickness WT_Params.Yaw_Actuator.yaw_ring_diameter/2*sin(1.0*pi)]$CG$CG$m$[0 0 0]$Euler X-Y-Z$deg$CG$false$none#Right$CS13$[WT_Params.Yaw_Actuator.yaw_ring_diameter/2*cos(1.2*pi) -0.5*WT_Params.Yaw_Actuator.yaw_ring_thickness WT_Params.Yaw_Actuator.yaw_ring_diameter/2*sin(1.2*pi)]$CG$CG$m$[0 0 0]$Euler X-Y-Z$deg$CG$false$none#Right$CS23$[WT_Params.Yaw_Actuator.yaw_ring_diameter/2*cos(1.2*pi) 0.5*WT_Params.Yaw_Actuator.yaw_ring_thickness WT_Params.Yaw_Actuator.yaw_ring_diameter/2*sin(1.2*pi)]$CG$CG$m$[0 0 0]$Euler X-Y-Z$deg$CG$false$none#Right$CS14$[WT_Params.Yaw_Actuator.yaw_ring_diameter/2*cos(1.4*pi) -0.5*WT_Params.Yaw_Actuator.yaw_gear_thickness WT_Params.Yaw_Actuator.yaw_ring_diameter/2*sin(1.4*pi)]$CG$CG$m$[0 0 0]$Euler X-Y-Z$deg$CG$false$none#Right$CS24$[WT_Params.Yaw_Actuator.yaw_ring_diameter/2*cos(1.4*pi) 0.5*WT_Params.Yaw_Actuator.yaw_ring_thickness WT_Params.Yaw_Actuator.yaw_ring_diameter/2*sin(1.4*pi)]$CG$CG$m$[0 0 0]$Euler X-Y-Z$deg$CG$false$none#Right$CS15$[WT_Params.Yaw_Actuator.yaw_ring_diameter/2*cos(1.6*pi) -0.5*WT_Params.Yaw_Actuator.yaw_ring_thickness WT_Params.Yaw_Actuator.yaw_ring_diameter/2*sin(1.6*pi)]$CG$CG$m$[0 0 0]$Euler X-Y-Z$deg$CG$false$none#Right$CS25$[WT_Params.Yaw_Actuator.yaw_ring_diameter/2*cos(1.6*pi) 0.5*WT_Params.Yaw_Actuator.yaw_ring_thickness WT_Params.Yaw_Actuator.yaw_ring_diameter/2*sin(1.6*pi)]$CG$CG$m$[0 0 0]$Euler X-Y-Z$deg$CG$false$none#Right$CS16$[WT_Params.Yaw_Actuator.yaw_ring_diameter/2*cos(1.8*pi) -0.5*WT_Params.Yaw_Actuator.yaw_ring_thickness WT_Params.Yaw_Actuator.yaw_ring_diameter/2*sin(1.8*pi)]$CG$CG$m$[0 0 0]$Euler X-Y-Z$deg$CG$false$none#Right$CS26$[WT_Params.Yaw_Actuator.yaw_ring_diameter/2*cos(1.8*pi) 0.5*WT_Params.Yaw_Actuator.yaw_ring_thickness WT_Params.Yaw_Actuator.yaw_ring_diameter/2*sin(1.8*pi)]$CG$CG$m$[0 0 0]$Euler X-Y-Z$deg$CG$false$none  CGPos=[0 0 0]  CGRot=[0 0 0]  CS0Pos=[]  CS0Rot=[]  CS1Pos=[0 0 0]  CS1Rot=[0 0 0]  CS2Pos=[0 0 0]  CS2Rot=[0 0 0]  CS3Pos=[0 0 0]  CS3Rot=[0 0 0]  CS4Pos=[0 0 0]  CS4Rot=[0 0 0]  CS5Pos=[0 0 0]  CS5Rot=[0 0 0]  CS6Pos=[0 0 0]  CS6Rot=[0 0 0]  CS7Pos=[WT_Params.Yaw_Actuator.yaw_ring_diameter/2*cos(0) -0.5*WT_Params.Yaw_Actuator.yaw_ring_thickness WT_Params.Yaw_Actuator.yaw_ring_diameter/2*sin(0)]  CS7Rot=[0 0 0]  CS8Pos=[WT_Params.Yaw_Actuator.yaw_ring_diameter/2*cos(0.2*pi) -0.5*WT_Params.Yaw_Actuator.yaw_gear_thickness WT_Params.Yaw_Actuator.yaw_ring_diameter/2*sin(0.2*pi)]  CS8Rot=[0 0 0]  CS9Pos=[WT_Params.Yaw_Actuator.yaw_ring_diameter/2*cos(0.4*pi) -0.5*WT_Params.Yaw_Actuator.yaw_ring_thickness WT_Params.Yaw_Actuator.yaw_ring_diameter/2*sin(0.4*pi)]  CS9Rot=[0 0 0]  CS10Pos=[WT_Params.Yaw_Actuator.yaw_ring_diameter/2*cos(0.6*pi) -0.5*WT_Params.Yaw_Actuator.yaw_ring_thickness WT_Params.Yaw_Actuator.yaw_ring_diameter/2*sin(0.6*pi)]  CS10Rot=[0 0 0]  CS11Pos=[WT_Params.Yaw_Actuator.yaw_ring_diameter/2*cos(0.8*pi) -0.5*WT_Params.Yaw_Actuator.yaw_ring_thickness WT_Params.Yaw_Actuator.yaw_ring_diameter/2*sin(0.8*pi)]  CS11Rot=[0 0 0]  CS12Pos=[WT_Params.Yaw_Actuator.yaw_ring_diameter/2*cos(1.0*pi) -0.5*WT_Params.Yaw_Actuator.yaw_ring_thickness WT_Params.Yaw_Actuator.yaw_gear_diameter/2*sin(1.0*pi)]  CS12Rot=[0 0 0]  CS13Pos=[WT_Params.Yaw_Actuator.yaw_ring_diameter/2*cos(1.2*pi) -0.5*WT_Params.Yaw_Actuator.yaw_ring_thickness WT_Params.Yaw_Actuator.yaw_ring_diameter/2*sin(1.2*pi)]  CS13Rot=[0 0 0]  CS14Pos=[WT_Params.Yaw_Actuator.yaw_ring_diameter/2*cos(1.4*pi) -0.5*WT_Params.Yaw_Actuator.yaw_gear_thickness WT_Params.Yaw_Actuator.yaw_ring_diameter/2*sin(1.4*pi)]  CS14Rot=[0 0 0]  CS15Pos=[WT_Params.Yaw_Actuator.yaw_ring_diameter/2*cos(1.6*pi) -0.5*WT_Params.Yaw_Actuator.yaw_ring_thickness WT_Params.Yaw_Actuator.yaw_ring_diameter/2*sin(1.6*pi)]  CS15Rot=[0 0 0]  CS16Pos=[WT_Params.Yaw_Actuator.yaw_ring_diameter/2*cos(1.8*pi) -0.5*WT_Params.Yaw_Actuator.yaw_ring_thickness WT_Params.Yaw_Actuator.yaw_ring_diameter/2*sin(1.8*pi)]  CS16Rot=[0 0 0]  CS17Pos=[WT_Params.Yaw_Actuator.yaw_ring_diameter/2*cos(0) 0.5*WT_Params.Yaw_Actuator.yaw_gear_thickness WT_Params.Yaw_Actuator.yaw_ring_diameter/2*sin(0)]  CS17Rot=[0 0 0]  CS18Pos=[WT_Params.Yaw_Actuator.yaw_ring_diameter/2*cos(0.2*pi) 0.5*WT_Params.Yaw_Actuator.yaw_ring_thickness WT_Params.Yaw_Actuator.yaw_ring_diameter/2*sin(0.2*pi)]  CS18Rot=[0 0 0]  CS19Pos=[WT_Params.Yaw_Actuator.yaw_ring_diameter/2*cos(0.4*pi) 0.5*WT_Params.Yaw_Actuator.yaw_ring_thickness WT_Params.Yaw_Actuator.yaw_ring_diameter/2*sin(0.4*pi)]  CS19Rot=[0 0 0]  CS20Pos=[WT_Params.Yaw_Actuator.yaw_ring_diameter/2*cos(0.6*pi) 0.5*WT_Params.Yaw_Actuator.yaw_ring_thickness WT_Params.Yaw_Actuator.yaw_ring_diameter/2*sin(0.6*pi)]  CS20Rot=[0 0 0]
  N1 : PMIOPort  Port=1  Side=Right
  N2 : PMIOPort  Port=2  Side=Right
  N : PMIOPort  Port=3  Side=Right
  N3 : PMIOPort  Port=4  Side=Right
  N4 : PMIOPort  Port=5  Side=Right
  T : PMIOPort  Port=6  Side=Left
  YC : PMIOPort  Port=7  Side=Right
  connections:
  T/RConn1 -- Yaw_Ring/RConn1
  Yaw_Ring/LConn4 -- Gear  Constraint3/LConn1
  Yaw_Ring/LConn2 -- Gear  Constraint2/LConn1
  Yaw_Ring/LConn1 -- Gear  Constraint1/LConn1
  Yaw_Ring/LConn3 -- Revolute/LConn1
  N/RConn1 -- Revolute/RConn1
  Nacelle Damping/LConn1 -- Revolute/LConn2
  Ideal Motor/RConn1 -- Rev_YG4/LConn2
  Ideal Motor/RConn2 -- Rev_YG3/LConn2
  Ideal Motor/RConn3 -- Rev_YG2/LConn2
  Ideal Motor/RConn4 -- Rev_YG1/LConn2
  YC/RConn1 -- Ideal Motor/LConn1
  Yaw Gear4/LConn1 -- Rev_YG4/LConn1
  Rev_YG4/RConn1 -- N4/RConn1
  Yaw_Ring/LConn5 -- Gear  Constraint4/LConn1
  Gear  Constraint4/RConn1 -- Yaw Gear4/RConn1
  Rev_YG3/RConn1 -- N3/RConn1
  Yaw Gear3/LConn1 -- Rev_YG3/LConn1
  Gear  Constraint3/RConn1 -- Yaw Gear3/RConn1
  Rev_YG2/RConn1 -- N2/RConn1
  Yaw Gear2/LConn1 -- Rev_YG2/LConn1
  Gear  Constraint2/RConn1 -- Yaw Gear2/RConn1
  N1/RConn1 -- Rev_YG1/RConn1
  Yaw Gear1/LConn1 -- Rev_YG1/LConn1
  Gear  Constraint1/RConn1 -- Yaw Gear1/RConn1

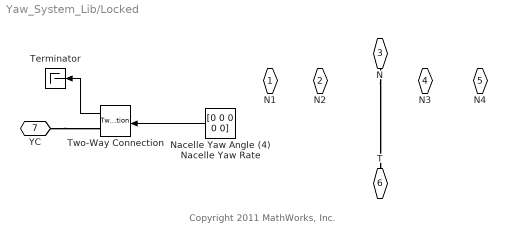
== system Yaw_System_Lib/Locked ==
  note: Copyright 2011 MathWorks, Inc.
  Nacelle Yaw Angle (4) Nacelle Yaw Rate : Constant  Value=[0 0 0 0 0]
  Terminator : Terminator
  Two-Way Connection : TwoWayConnection
  N1 : PMIOPort  Port=1  Side=Right
  N2 : PMIOPort  Port=2  Side=Right
  N : PMIOPort  Port=3  Side=Right
  N3 : PMIOPort  Port=4  Side=Right
  N4 : PMIOPort  Port=5  Side=Right
  T : PMIOPort  Port=6  Side=Left
  YC : PMIOPort  Port=7  Side=Right
  wires:
  Nacelle Yaw Angle (4) Nacelle Yaw Rate/1 -> Two-Way Connection/1
  Two-Way Connection/1 -> Terminator/1
  connections:
  N/RConn1 -- T/RConn1
  YC/RConn1 -- Two-Way Connection/RConn1
